simulink model "QRsim"  (R2013b)
settings: Solver=ode45  StartTime=0.0  StopTime=10.0  RelTol=1e-3
undefined symbols (not defined in the file): b, d, g, Ixx, Iyy, Izz, Jr, l, m, phi0, phidot0, psi0, psidot0, theta0, thetadot0, x0, xdot0, y0, ydot0, z0, zdot0
settings Model: Creator=Nam  LastModifiedBy=Nam

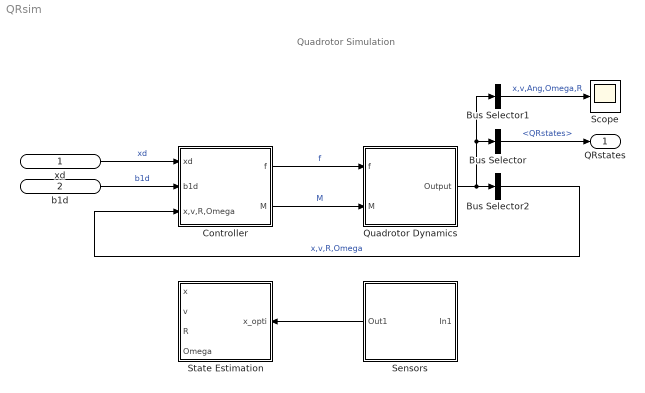
== system QRsim ==
  note: Quadrotor Simulation
  xd : Inport
  b1d : Inport  Port=2
  Bus Selector : BusSelector  OutputSignals=QRstates
  Bus Selector1 : BusSelector  OutputSignals=QROutput.x,QROutput.v,QROutput.Ang,QROutput.Omega,QROutput.R  OutputAsBus=on
  Bus Selector2 : BusSelector  OutputSignals=QROutput.x,QROutput.v,QROutput.R,QROutput.Omega  OutputAsBus=on
  Controller : Subsystem
      mask Display: disp('Controller')
  Quadrotor Dynamics : Subsystem
      mask Display: image('bebop.png')
  Scope : Scope
  Sensors : Subsystem
      mask Display: image('optitrack.jpg')
  State Estimation : Subsystem
  QRstates : Outport
  wires:
  Sensors/1(Out1) -> State Estimation/1(x_opti)
  xd/1 -> Controller/1(xd)  "xd"
  b1d/1 -> Controller/2(b1d)  "b1d"
  Controller/1(f) -> Quadrotor Dynamics/1(f)  "f"
  Controller/2(M) -> Quadrotor Dynamics/2(M)  "M"
  Bus Selector/1 -> QRstates/1  "<QRstates>"
  Bus Selector1/1 -> Scope/1  "x,v,Ang,Omega,R"
  Bus Selector2/1 -> Controller/3(x,v,R,Omega)  "x,v,R,Omega"
  Quadrotor Dynamics/1(Output) -> Bus Selector/1, Bus Selector1/1, Bus Selector2/1

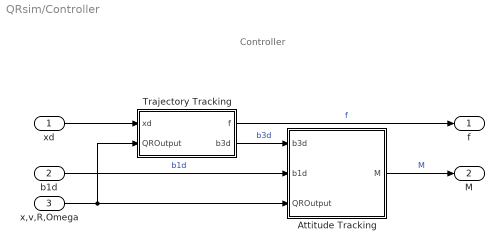
== system QRsim/Controller ==
  note: Controller
  xd : Inport
  b1d : Inport  Port=2
  x,v,R,Omega : Inport  Port=3
  Attitude Tracking : Subsystem
      mask Display: disp('Attitude\nTracking')
  Trajectory Tracking : Subsystem
      mask Display: disp('Trajectory\nTracking')
  f : Outport
  M : Outport  Port=2
  wires:
  b1d/1 -> Attitude Tracking/2(b1d)  "b1d"
  Trajectory Tracking/1(f) -> f/1  "f"
  Attitude Tracking/1(M) -> M/1  "M"
  x,v,R,Omega/1 -> Attitude Tracking/3(QROutput), Trajectory Tracking/2(QROutput)
  xd/1 -> Trajectory Tracking/1(xd)
  Trajectory Tracking/2(b3d) -> Attitude Tracking/1(b3d)  "b3d"

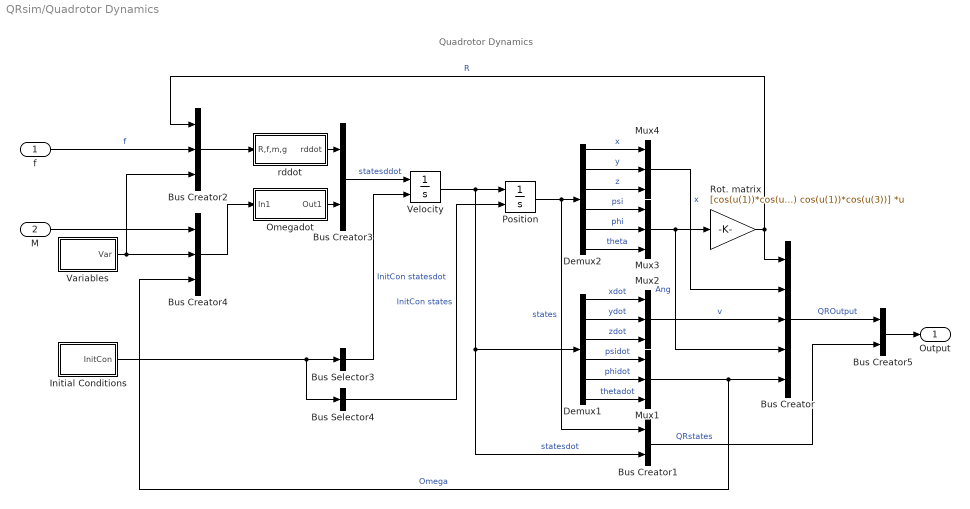
== system QRsim/Quadrotor Dynamics ==
  note: Quadrotor Dynamics
  f : Inport
  M : Inport  Port=2
  Bus Creator : BusCreator  Inputs=5
  Bus Creator1 : BusCreator  Inputs=2
  Bus Creator2 : BusCreator  Inputs=3
  Bus Creator3 : BusCreator  Inputs=2
  Bus Creator4 : BusCreator  Inputs=3
  Bus Creator5 : BusCreator  Inputs=2
  Bus Selector3 : BusSelector  OutputSignals=InitCon dot.x0,InitCon dot.y0,InitCon dot.z0,InitCon dot.psi0,InitCon dot.phi0,InitCon dot.theta0  OutputAsBus=on
  Bus Selector4 : BusSelector  OutputSignals=InitCon.x0,InitCon.y0,InitCon.z0,InitCon.psi0,InitCon.phi0,InitCon.theta0  OutputAsBus=on
  Demux1 : Demux  Outputs=6
  Demux2 : Demux  Outputs=6
  Initial Conditions : Subsystem
      mask Display: disp('Initial\nConditions')
  Mux{1..4} (4 alike) : Mux  Inputs=3
  Omegadot : Subsystem
      mask Display: disp('[\psi{"}; \phi{"}; \theta{"}]','texmode','on')
  Position : Integrator  InitialConditionSource=external
  Rot. matrix : Gain  Gain=|  Multiplication=Matrix(K*u)
      | [cos(u(1))*cos(u(3))-sin(u(2))*sin(u(1))*sin(u(3)) -cos(u(3))*sin(u(1)) cos(u(1))*sin(u(3))+cos(u(3))*sin(u(2))*sin(u(1));
      | cos(u(3))*sin(u(1))+cos(u(1))*sin(u(2))*sin(u(3)) cos(u(1))*cos(u(3)) sin(u(1))*sin(u(3))-cos(u(1))*cos(u(3))*sin(u(2));
      | -cos(u(2))*sin(u(3)) sin(u(1)) cos(u(1))*cos(u(3))]
      mask Display: disp('R(\psi,\phi,\theta)','texmode','on')
  Variables : Subsystem
      mask Display: disp('Variables')
  Velocity : Integrator  InitialConditionSource=external
  rddot : Subsystem
      mask Display: disp('[x{"}; y{"}; z{"}]','texmode','on')
  Output : Outport
  wires:
  Velocity/1 -> Position/1, Bus Creator1/2, Demux1/1  "statesdot"
  f/1 -> Bus Creator2/2  "f"
  Variables/1(Var) -> Bus Creator4/2, Bus Creator2/3
  Bus Creator2/1 -> rddot/1(R,f,m,g)
  M/1 -> Bus Creator4/1
  Position/1 -> Bus Creator1/1, Demux2/1  "states"
  Rot. matrix/1 -> Bus Creator2/1, Bus Creator/1  "R"
  Mux1/1 -> Bus Creator4/3, Bus Creator/5  "Omega"
  rddot/1(rddot) -> Bus Creator3/1
  Bus Creator3/1 -> Velocity/1  "statesddot"
  Initial Conditions/1(InitCon) -> Bus Selector3/1, Bus Selector4/1
  Bus Selector3/1 -> Velocity/2  "InitCon statesdot"
  Bus Selector4/1 -> Position/2  "InitCon states"
  Omegadot/1(Out1) -> Bus Creator3/2
  Bus Creator4/1 -> Omegadot/1(In1)
  Demux1/4 -> Mux1/1  "psidot"
  Demux1/5 -> Mux1/2  "phidot"
  Demux1/6 -> Mux1/3  "thetadot"
  Demux1/2 -> Mux2/2  "ydot"
  Demux1/1 -> Mux2/1  "xdot"
  Demux1/3 -> Mux2/3  "zdot"
  Mux2/1 -> Bus Creator/3  "v"
  Demux2/4 -> Mux3/1  "psi"
  Demux2/5 -> Mux3/2  "phi"
  Demux2/6 -> Mux3/3  "theta"
  Demux2/2 -> Mux4/2  "y"
  Demux2/1 -> Mux4/1  "x"
  Demux2/3 -> Mux4/3  "z"
  Mux3/1 -> Bus Creator/4, Rot. matrix/1  "Ang"
  Mux4/1 -> Bus Creator/2  "x"
  Bus Creator/1 -> Bus Creator5/1  "QROutput"
  Bus Creator1/1 -> Bus Creator5/2  "QRstates"
  Bus Creator5/1 -> Output/1

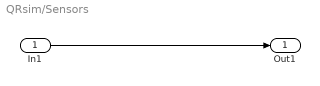
== system QRsim/Sensors ==
  In1 : Inport
  Out1 : Outport
  wires:
  In1/1 -> Out1/1

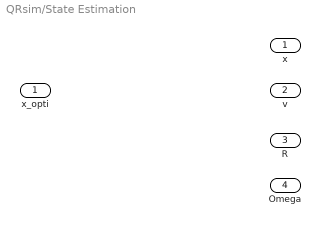
== system QRsim/State Estimation ==
  x_opti : Inport
  x : Outport
  v : Outport  Port=2
  R : Outport  Port=3
  Omega : Outport  Port=4

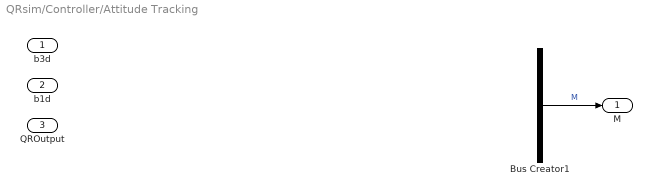
== system QRsim/Controller/Attitude Tracking ==
  b3d : Inport
  b1d : Inport  Port=2
  QROutput : Inport  Port=3
  Bus Creator1 : BusCreator  Inputs=3
  M : Outport
  wires:
  Bus Creator1/1 -> M/1  "M"

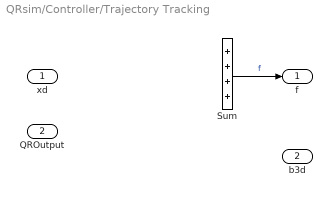
== system QRsim/Controller/Trajectory Tracking ==
  xd : Inport
  QROutput : Inport  Port=2
  Sum : Sum  Inputs=++++
  f : Outport
  b3d : Outport  Port=2
  wires:
  Sum/1 -> f/1  "f"

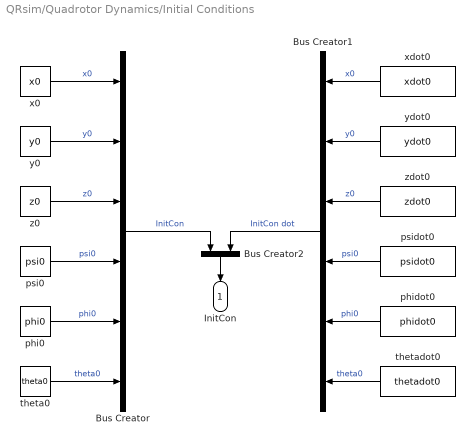
== system QRsim/Quadrotor Dynamics/Initial Conditions ==
  Bus Creator : BusCreator  Inputs=6
  Bus Creator1 : BusCreator  Inputs=6
  Bus Creator2 : BusCreator  Inputs=2
  phi0 : Constant  Value=phi0
  phidot0 : Constant  Value=phidot0
  psi0 : Constant  Value=psi0
  psidot0 : Constant  Value=psidot0
  theta0 : Constant  Value=theta0
  thetadot0 : Constant  Value=thetadot0
  x0 : Constant  Value=x0
  xdot0 : Constant  Value=xdot0
  y0 : Constant  Value=y0
  ydot0 : Constant  Value=ydot0
  z0 : Constant  Value=z0
  zdot0 : Constant  Value=zdot0
  InitCon : Outport
  wires:
  phi0/1 -> Bus Creator/5  "phi0"
  y0/1 -> Bus Creator/2  "y0"
  psi0/1 -> Bus Creator/4  "psi0"
  x0/1 -> Bus Creator/1  "x0"
  z0/1 -> Bus Creator/3  "z0"
  theta0/1 -> Bus Creator/6  "theta0"
  Bus Creator1/1 -> Bus Creator2/2  "InitCon dot"
  psidot0/1 -> Bus Creator1/4  "psi0"
  xdot0/1 -> Bus Creator1/1  "x0"
  zdot0/1 -> Bus Creator1/3  "z0"
  ydot0/1 -> Bus Creator1/2  "y0"
  phidot0/1 -> Bus Creator1/5  "phi0"
  thetadot0/1 -> Bus Creator1/6  "theta0"
  Bus Creator2/1 -> InitCon/1
  Bus Creator/1 -> Bus Creator2/1  "InitCon"

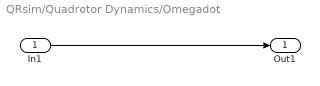
== system QRsim/Quadrotor Dynamics/Omegadot ==
  In1 : Inport
  Out1 : Outport
  wires:
  In1/1 -> Out1/1

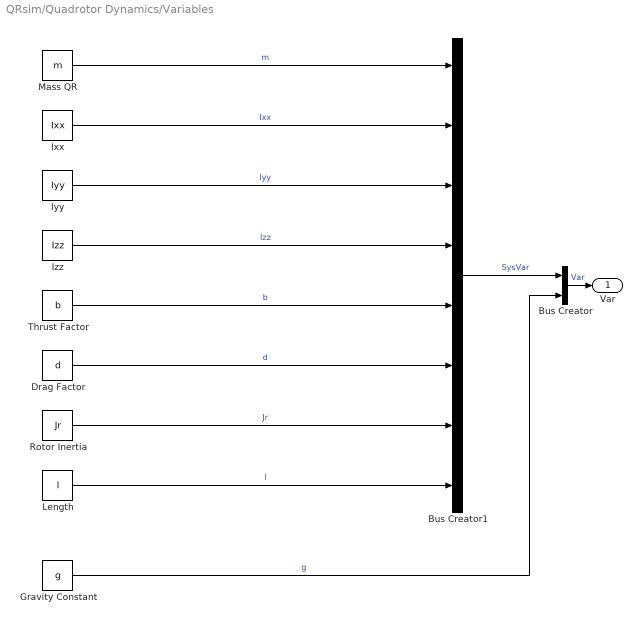
== system QRsim/Quadrotor Dynamics/Variables ==
  Bus Creator : BusCreator  Inputs=2
  Bus Creator1 : BusCreator  Inputs=8
  Drag Factor : Constant  Value=d
  Gravity Constant : Constant  Value=g
  Ixx : Constant  Value=Ixx
  Iyy : Constant  Value=Iyy
  Izz : Constant  Value=Izz
  Length : Constant  Value=l
  Mass QR : Constant  Value=m
  Rotor Inertia : Constant  Value=Jr
  Thrust Factor : Constant  Value=b
  Var : Outport
  wires:
  Gravity Constant/1 -> Bus Creator/2  "g"
  Bus Creator/1 -> Var/1  "Var"
  Izz/1 -> Bus Creator1/4  "Izz"
  Mass QR/1 -> Bus Creator1/1  "m"
  Drag Factor/1 -> Bus Creator1/6  "d"
  Iyy/1 -> Bus Creator1/3  "Iyy"
  Length/1 -> Bus Creator1/8  "l"
  Rotor Inertia/1 -> Bus Creator1/7  "Jr"
  Thrust Factor/1 -> Bus Creator1/5  "b"
  Ixx/1 -> Bus Creator1/2  "Ixx"
  Bus Creator1/1 -> Bus Creator/1  "SysVar"

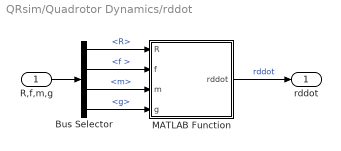
== system QRsim/Quadrotor Dynamics/rddot ==
  R,f,m,g : Inport
  Bus Selector : BusSelector  OutputSignals=R,f ,Var.SysVar.m,Var.g
  MATLAB Function : MATLAB Function  TreatAsAtomicUnit=on
  rddot : Outport
  wires:
  R,f,m,g/1 -> Bus Selector/1
  Bus Selector/1 -> MATLAB Function/1(R)  "<R>"
  MATLAB Function/1(rddot) -> rddot/1  "rddot"
  Bus Selector/3 -> MATLAB Function/3(m)  "<m>"
  Bus Selector/4 -> MATLAB Function/4(g)  "<g>"
  Bus Selector/2 -> MATLAB Function/2(f)  "<f >"

== matlab function QRsim/Quadrotor Dynamics/rddot/MATLAB Function ==
  data: R input; rddot output; f input; m input; g input
function rddot = fcn(R,f,m,g)
%rddot = [xddot; yddot; zddot]
%e3 downwards

[rddot] = g*[0;0;1]-f/m*R*[0;0;1];
